simulink model "TV_render_car"  (R2025b)
settings: Solver=VariableStepAuto  StartTime=0.0  StopTime=90  MaxStep=0.03  RelTol=1e-3
libraries: simulink x4, vehdynlibsteering x1, sim3dlib x1, sim3dautolib x1, slpidlib x1, autolibshared x1
settings Model: Creator=Utente  LastModifiedBy=Utente

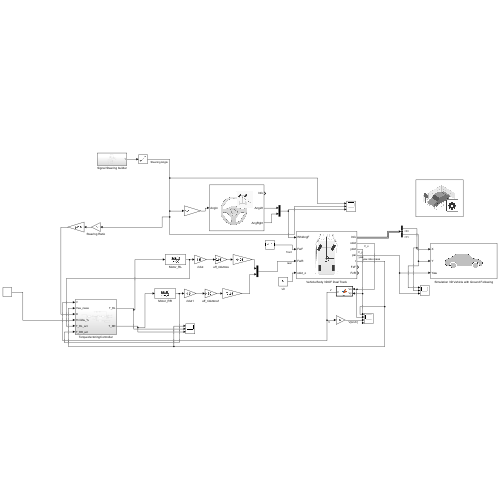
[thumbnail: Simulink's stored preview of the top-level diagram]
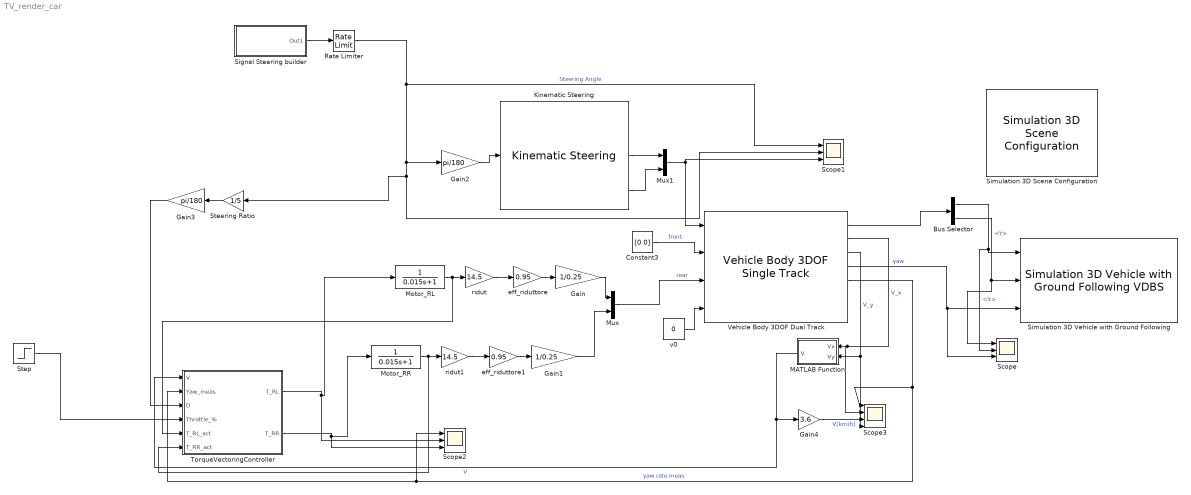
== system TV_render_car ==
  Bus Selector : BusSelector  OutputSignals=InertFrm.Geom.Disp.X,InertFrm.Geom.Disp.Y
  Constant3 : Constant  Value=[0 0]
  Gain : Gain  Gain=1/0.25
  Gain1 : Gain  Gain=1/0.25
  Gain2 : Gain  Gain=pi/180
  Gain3 : Gain  Gain=pi/180
  Gain4 : Gain  Gain=3.6
  Kinematic Steering : vehdynlibsteering/Kinematic Steering  StrgType=Ackerman  StrgRatioType=Constant  Loc=Front  NrmlFctr=0.01  TrckWdth=1.2  WhlBase=1.55  Db=0  StrgRng=pi  StrgAngBpts="[-6.2832   -5.0265   -3.7699   -2.5133   -1.2566         0    1.2566    2.5133    3.7699    5.0265    6.2832]"  StrgRatioTbl=|  StrgRatio=5  PctAckIn=off  PctAck=100  PctAckTbl=ones(1,11)*100  StrgArmLngth=0.1  RckCsLngth=0.5  TieRodLngth=0.248  D=0.2  PnnRadius=0.00085818  PnnRadiusTbl="[0.0055    0.0055    0.0056    0.0057    0.0058    0.0057    0.0057    0.0057    0.0056    0.0055    0.0055]"  RodLngth=0.1  ParaArmLngth=0.9  aMode=2
      | [13.5000   13.3750   13.2500   13.1250   13.0000   13.0000   13.0000   13.1250   13.2500   13.3750   13.5000
      | ]
  MATLAB Function : MATLAB Function  TreatAsAtomicUnit=on
  Motor_RL : TransferFcn  Denominator=[0.015 1]
  Motor_RR : TransferFcn  Denominator=[0.015 1]
  Mux : Mux  Inputs=2
  Mux1 : Mux  Inputs=2
  Rate Limiter : RateLimiter  RisingSlewLimit=300  FallingSlewLimit=-300  SampleTimeMode=inherited
  Scope : Scope  NumInputPorts=3
      settings: ActiveDisplayYMinimum=-522.68712025168293  ActiveDisplayYMaximum=261.84287437072271
  Scope1 : Scope  NumInputPorts=3
      settings: ActiveDisplayYMinimum=-50  ActiveDisplayYMaximum=50
  Scope2 : Scope  NumInputPorts=3
      settings: ActiveDisplayYMinimum=-1.4348752582042583  ActiveDisplayYMaximum=1.2936169370543145  DataLoggingVariableName=ScopeData2
  Scope3 : Scope  NumInputPorts=4
      settings: ActiveDisplayYMinimum=-15.9041702308022  ActiveDisplayYMaximum=143.13753207721982  DataLoggingVariableName=ScopeData3
  Signal Steering builder : Subsystem
  Simulation 3D Scene Configuration : sim3dlib/Simulation 3D Scene Configuration  Priority=0  ProjectFormat=Default Scenes  SceneDesc=Double lane change  ProjectName=Z:\.Programmi\MATLAB\toolbox\shared\sim3d_projects\automotive_project_windows\UE\WindowsNoEditor\VehicleSimulation.exe  ScenePath=/Game/Maps/HwStrght  EnableOpenDRIVE=off  vehTagList={'Custom';'Scene Origin';'SimulinkVehicle1'}  vehTag=SimulinkVehicle1  AttachedCameraRelativeTranslation=[0 0 0]  FreeCameraDefaultInitialTranslation=[-6, 0, 2]  AttachedCameraRelativeRotation=[0 0 0]  FreeCameraDefaultInitialRotation=[0, -15, 0]  ViewpointName=Custom  FreeCameraInitialTranslation=[0 0 0]  ViewpointTranslation=[0 0 0]  FreeCameraInitialRotation=[0 0 0]  ViewpointRotation=[0 0 0]  OpVisEn=off  Ts=.02  EnableWindow=on  EnableRemoteAccess=off  EnableWeather=off  SunAzimuth=90  SunAltitude=40.0  EnableGeospatialSun=off  Latitude=0  Longitude=0  Date=2023-01-01  Time=10:30:00  GeoTimeZone=-5.0  SunDaylightSaving=off  wind=1  clouds=10  EnableVolumetricClouds=off  CloudCoverage=0  CloudAltitude=6  fog=0  rain=0  RaindropsEffect=off  SnowDensity=0  EnableGeospatial=off  TilesetSource=Earth terrain  UseTrueOrigin=off  OriginHeight=200  OriginLatitude=40.744652  OriginLongitude=-73.988864  MapStyle=Aerial  AdditionalAssetIDs=[]  UseAdvancedSunSky=off  SolarTime=11  TimeZone=-5  Day=21  Month=9  Year=2022  UseDaylightSavingTime=on  DSTStartDay=10  DSTStartMonth=3  DSTEndDay=3  DSTEndMonth=11  DSTSwitchHour=2  sensorTag=MainCamera1  sensorId=1  sensorName=MainCamera1  mountLoc=Origin  offsetFlag=off  tmountOffset=[0, 0, 0]  rmountOffset=[0, 0, 0]  HorizontalResolution=1280  VerticalResolution=720  HorizontalFOV=60  mountPoint=[0 0 0]  mountOrientation=[0 0 0]  aMode=2  ID=1  GeoTrigger=Inactive  ViewNameList={'Custom'}  ViewTranslationList={'[0 0 0]'}  ViewRotationList={'[0 0 0]'}
      settings: LibrarySourceBlock=vehdynlibsim3dcore/Simulation 3D Scene Configuration
  Simulation 3D Vehicle with Ground Following : sim3dautolib/Simulation 3D Vehicle with Ground Following VDBS  Priority=-1  PassVehMesh=Formula student vehicle  MeshPath=/MathWorksAutomotiveContent/Vehicles/Muscle/Meshes/SK_MuscleCar.SK_MuscleCar  TrackWidth=1.9  WheelBase=3  WheelRadius=0.35  VehColor=Red  CoordinateSystem=SAE  InitialPos=[0, 0, 0]  InitialRot=[0,0,0]  ActorName=SimulinkVehicle1  VehLightsControl=off  HeadlightColor=[ 1, 1, 1 ]  HighBeamIntensity=100000  LowBeamIntensity=60000  HighBeamConeAngle=1.22  LowBeamConeAngle=1.22  LeftHeadlightOrientation=[ 0, 0 ]  RightHeadlightOrientation=[ 0, 0 ]  BrakelightIntensity=200  ReverselightIntensity=500  SignallightIntensity=500  SignallightPeriod=1  SignalPulseWidth=50  SampleTime=-1  ActorType=SimulinkVehicle  ID=1  aMode=2  ActorTag=SimulinkVehicle1  CoordinateScheme=0
      settings: LibrarySourceBlock=vehdynlibsim3d/Simulation 3D Vehicle with Ground Following
  Steering Ratio : Gain  Gain=1/5
  Step : Step  Time=2  After=50  SampleTime=0
  TorqueVectoringController : Subsystem
  Vehicle Body 3DOF Dual Track : autolibshared/Vehicle Body 3DOF Single Track  trackMode=Dual  inputMode=External longitudinal forces  frontSteerMode=on  rearSteerMode=off  windMode=off  muMode=off  extFMode=off  extMMode=off  htchFMode=off  htchMMode=off  extXo=off  extpsio=off  extxdoto=on  extro=off  extYo=off  extTamb=off  extydoto=off  aMode=2  NF=2  NR=2  m=320  a=0.775  b=0.775  h=0.35  dh=1  hh=0.2  X_o=0  xdot_o=0  CalphaMode=off  sigmaMode=on  d=0  hl=0  w=[1.2,1.2]  Cy_f=35e3  Cy_r=45e3  sigma_f=.1  sigma_r=.1  alpha_f_brk=[-0.785, -0.628, -0.471, -0.314, -0.157, 0.000, 0.157, 0.314, 0.471, 0.628, 0.785]  Cy_f_data=[2000, 3000, 4000, 5500, 7000, 9000, 7000, 5500, 4000, 3000, 2000]  alpha_r_brk=[-0.785, -0.628, -0.471, -0.314, -0.157, 0.000, 0.157, 0.314, 0.471, 0.628, 0.785]  Cy_r_data=[2000, 3000, 4000, 5500, 7000, 9000, 7000, 5500, 4000, 3000, 2000]  Y_o=5  ydot_o=0  Izz=200  psi_o=0  r_o=0  Af=1.1  Cd=1.3  Cl=-1  Cpm=.1  beta_w=[0 0.01:0.01:0.3]  Cs=[0:0.03:0.9]  Cym=[0 1e-6:0.01:0.3]  Pabs=101325  Tair=273  g=9.81  mu=1  xdot_tol=.01  Fznom=2400  Fxtire_sat=7e4  Fytire_sat=7e4  longOff=0  latOff=0  vertOff=0  wrapAng=off
      settings: LibrarySourceBlock=vehdynlibeom/Vehicle Body 3DOF Dual Track
  eff_riduttore : Gain  Gain=0.95
  eff_riduttore1 : Gain  Gain=0.95
  ridut : Gain  Gain=14.5
  ridut1 : Gain  Gain=14.5
  v0 : Constant  Value=0
  wires:
  Constant3/1 -> Vehicle Body 3DOF Dual Track/2  "front"
  Mux/1 -> Vehicle Body 3DOF Dual Track/3  "rear"
  Gain/1 -> Mux/1
  Gain1/1 -> Mux/2
  Kinematic Steering/2 -> Mux1/1
  Kinematic Steering/3 -> Mux1/2
  Mux1/1 -> Vehicle Body 3DOF Dual Track/1, Scope1/3
  Gain2/1 -> Kinematic Steering/1
  Vehicle Body 3DOF Dual Track/2 -> Scope3/2, MATLAB Function/1(Vx)  "V_x"
  Vehicle Body 3DOF Dual Track/3 -> Scope3/4, MATLAB Function/2(Vy)  "V_y"
  Bus Selector/1 -> Scope/2, Simulation 3D Vehicle with Ground Following/1  "<X>"
  Bus Selector/2 -> Scope/1, Simulation 3D Vehicle with Ground Following/2  "<Y>"
  Vehicle Body 3DOF Dual Track/5 -> Scope2/1, TorqueVectoringController/2(Yaw_meas), Scope3/1  "yaw rate meas"
  v0/1 -> Vehicle Body 3DOF Dual Track/4
  Vehicle Body 3DOF Dual Track/1 -> Bus Selector/1
  Motor_RL/1 -> TorqueVectoringController/5(T_RL_act), ridut/1
  eff_riduttore/1 -> Gain/1
  ridut/1 -> eff_riduttore/1
  Motor_RR/1 -> TorqueVectoringController/6(T_RR_act), ridut1/1
  ridut1/1 -> eff_riduttore1/1
  eff_riduttore1/1 -> Gain1/1
  Steering Ratio/1 -> Gain3/1
  Gain3/1 -> TorqueVectoringController/3(D)
  Step/1 -> TorqueVectoringController/4(Throttle_%)
  MATLAB Function/1(V) -> TorqueVectoringController/1(V), Gain4/1  "V"
  Vehicle Body 3DOF Dual Track/4 -> Scope/3, Simulation 3D Vehicle with Ground Following/3  "yaw"
  Signal Steering builder/1(Out1) -> Rate Limiter/1
  TorqueVectoringController/1(T_RL) -> Scope2/2, Motor_RL/1
  TorqueVectoringController/2(T_RR) -> Scope2/3, Motor_RR/1
  Gain4/1 -> Scope3/3  "V[km/h]"
  Rate Limiter/1 -> Steering Ratio/1, Scope1/2, Gain2/1, Scope1/1  "Steering Angle"

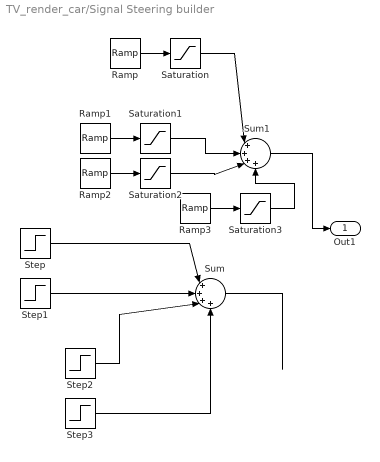
== system TV_render_car/Signal Steering builder ==
  Ramp : simulink/Sources/Ramp  slope=20  start=0  InitialOutput=0
  Ramp1 : simulink/Sources/Ramp  slope=-20  start=14  InitialOutput=0
  Ramp2 : simulink/Sources/Ramp  slope=-20  start=14  InitialOutput=0
  Ramp3 : simulink/Sources/Ramp  slope=20  start=22  InitialOutput=0
  Saturation{,1..3} (4 alike) : Saturate  UpperLimit=40  LowerLimit=-40
  Step : Step  Time=6  After=50  SampleTime=0
  Step1 : Step  Time=14  After=-50  SampleTime=0
  Step2 : Step  Time=14  After=-50  SampleTime=0
  Step3 : Step  Time=22  After=50  SampleTime=0
  Sum : Sum  Inputs=|++++
  Sum1 : Sum  Inputs=|++++
  Out1 : Outport
  wires:
  Step/1 -> Sum/1
  Step1/1 -> Sum/2
  Step3/1 -> Sum/4
  Step2/1 -> Sum/3
  Sum/1 -> ?
  Ramp/1 -> Saturation/1
  Ramp1/1 -> Saturation1/1
  Ramp2/1 -> Saturation2/1
  Ramp3/1 -> Saturation3/1
  Saturation3/1 -> Sum1/4
  Saturation/1 -> Sum1/1
  Saturation1/1 -> Sum1/2
  Saturation2/1 -> Sum1/3
  Sum1/1 -> Out1/1

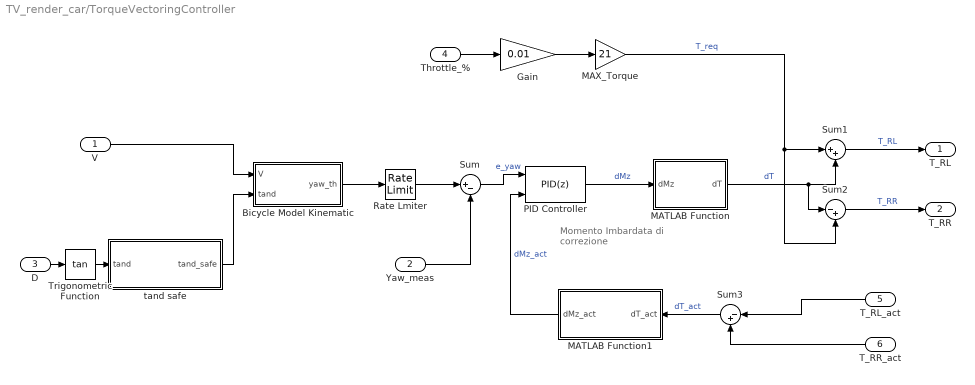
== system TV_render_car/TorqueVectoringController ==
  note: Momento Imbardata di correzione
  V : Inport
  Yaw_meas : Inport  Port=2
  D : Inport  Port=3
  Throttle_% : Inport  Port=4
  T_RL_act : Inport  Port=5
  T_RR_act : Inport  Port=6
  Bicycle Model Kinematic : MATLAB Function  TreatAsAtomicUnit=on
  Gain : Gain  Gain=0.01
  MATLAB Function : MATLAB Function  TreatAsAtomicUnit=on
  MATLAB Function1 : MATLAB Function  TreatAsAtomicUnit=on
  MAX_Torque : Gain  Gain=21
  PID Controller : slpidlib/PID Controller  Controller=PID  Form=Parallel  TimeDomain=Discrete-time  UseExternalTs=off  SampleTime=0.05  IntegratorMethod=Forward Euler  FilterMethod=Forward Euler  ControllerParametersSource=internal  P=50  I=0.01  UseKiTs=off  D=0  UseExternalDerivativeSource=off  N=100  UseFilter=on  TunerSelectOption=Transfer Function Based (PID Tuner App)  InitialConditionSource=internal  InitialConditionForIntegrator=0  InitialConditionForFilter=0  DifferentiatorICPrevScaledInput=0  ExternalReset=none  TrackingMode=on  Kt=0.7  LimitOutput=on  SatLimitsSource=internal  UpperSaturationLimit=10  LowerSaturationLimit=-10  LinearizeAsGain=on  AntiWindupMode=none  Kb=1  LimitIntegrator=off  UpperIntegratorSaturationLimit=inf  LowerIntegratorSaturationLimit=-inf  POutMin=[]  POutMax=[]  IOutMin=[]  IOutMax=[]  DOutMin=[]  DOutMax=[]  NOutMin=[]  NOutMax=[]  SumOutMin=[]  SumOutMax=[]  SaturationOutMin=[]  SaturationOutMax=[]  PParamMin=[]  PParamMax=[]  IParamMin=[]  IParamMax=[]  DParamMin=[]  DParamMax=[]  NParamMin=[]  NParamMax=[]  KbParamMin=[]  KbParamMax=[]  KtParamMin=[]  KtParamMax=[]  KbOutMin=[]  KbOutMax=[]  KtOutMin=[]  KtOutMax=[]  IntegratorOutMin=[]  IntegratorOutMax=[]  FilterOutMin=[]  FilterOutMax=[]  SumI1OutMin=[]  SumI1OutMax=[]  SumI2OutMin=[]  SumI2OutMax=[]  SumI3OutMin=[]  SumI3OutMax=[]  SumI4OutMin=[]  SumI4OutMax=[]  SumDOutMin=[]  SumDOutMax=[]  DifferentiatorOutMin=[]  DifferentiatorOutMax=[]  FilterDiffOutCoefMin=[]  FilterDiffOutCoefMax=[]  ReciprocalOutMin=[]  ReciprocalOutMax=[]  SumDenOutMin=[]  SumDenOutMax=[]  SumNumOutMin=[]  SumNumOutMax=[]  DivideOutMin=[]  DivideOutMax=[]  UdiffTsProdOutMin=[]  UdiffTsProdOutMax=[]  NTsProdOutMin=[]  NTsProdOutMax=[]  UintegralTsProdOutMin=[]  UintegralTsProdOutMax=[]  UngainTsProdOutMin=[]  UngainTsProdOutMax=[]  ClampingZeroOutDataTypeStr=Inherit: Inherit via back propagation  ClampingZeroOutMin=[]  ClampingZeroOutMax=[]  FilterDenConstantOutDataTypeStr=Inherit: Inherit via back propagation  FilterDenConstantOutMin=[]  FilterDenConstantOutMax=[]  PCopyOutDataTypeStr=Inherit: Inherit via back propagation  PCopyOutMin=[]  PCopyOutMax=[]  NCopyOutDataTypeStr=Inherit: Inherit via back propagation  NCopyOutMin=[]  NCopyOutMax=[]  IntegratorContinuousStateAttributes=''  IntegratorStateMustResolveToSignalObject=off  IntegratorRTWStateStorageClass=Auto  FilterContinuousStateAttributes=''  FilterStateMustResolveToSignalObject=off  FilterRTWStateStorageClass=Auto  ParallelPVariant=InternalParameters  IdealPVariant=Disabled  IVariant=InternalParameters  DVariant=InternalParameters  IntegratorVariant=Discrete  SatVariant=Enabled  AWVariant=Passthrough  PCopyVariant=Disabled  TRVariant=Enabled  FdbkBlocksVariant=Forward  IdealPFdbkVariant=Disabled  SatFdbkVariant=Disabled  DerivativeFilterVariant=ForwardEulerFilter  NVariant=InternalParameters  NCopyVariant=Disabled  FilterICVariant=InternalICsFilter  IntegratorICVariant=InternalICs  ExternalResetVariant=Disabled  TRSumVariant=TrackingMode  SumFdbkVariant=Disabled  SumVariant=Sum_PID  TsampFilterVariant=InternalTs  TsampNgainVariant=Passthrough  TsampIntegralVariant=Disabled_SignalSpec  ExternalSaturationOutDataTypeStr=Inherit: Same as second input  DerivativeSourceVariant=ErrorSignal  PreIntVariant=InternalPreInt
  Rate Lmiter : RateLimiter  RisingSlewLimit=0.5  FallingSlewLimit=-0.5  SampleTimeMode=inherited
  Sum : Sum  Inputs=|+-
  Sum1 : Sum  Inputs=|++
  Sum2 : Sum  Inputs=|-+
  Sum3 : Sum  Inputs=|-+
  Trigonometric Function : Trigonometry  Operator=tan
  tand safe : MATLAB Function  TreatAsAtomicUnit=on
  T_RL : Outport
  T_RR : Outport  Port=2
  wires:
  Throttle_%/1 -> Gain/1
  Trigonometric Function/1 -> tand safe/1(tand)
  D/1 -> Trigonometric Function/1
  tand safe/1(tand_safe) -> Bicycle Model Kinematic/2(tand)
  V/1 -> Bicycle Model Kinematic/1(V)
  Yaw_meas/1 -> Sum/2
  Sum/1 -> PID Controller/1  "e_yaw"
  PID Controller/1 -> MATLAB Function/1(dMz)  "dMz"
  MAX_Torque/1 -> Sum2/2, Sum1/1  "T_req"
  Sum1/1 -> T_RL/1  "T_RL"
  MATLAB Function/1(dT) -> Sum2/1, Sum1/2  "dT"
  Sum2/1 -> T_RR/1  "T_RR"
  Sum3/1 -> MATLAB Function1/1(dT_act)  "dT_act"
  MATLAB Function1/1(dMz_act) -> PID Controller/2  "dMz_act"
  Gain/1 -> MAX_Torque/1
  T_RL_act/1 -> Sum3/1
  T_RR_act/1 -> Sum3/2
  Bicycle Model Kinematic/1(yaw_th) -> Rate Lmiter/1
  Rate Lmiter/1 -> Sum/1

== matlab function TV_render_car/TorqueVectoringController/Bicycle Model Kinematic ==
  data: V input; yaw_th output; tand input
function yaw_th = fcn(V,tand)
L = 1.55; %passo veicolo [m]
yaw_th = (V / L) * tand;

== matlab function TV_render_car/TorqueVectoringController/MATLAB Function1 ==
  data: dT_act input; dMz_act output
function dMz_act = fcn(dT_act)
Rw = 0.2; %raggio ruota [m]
w  = 1.2; %carreggiata [m]

dMz_act = dT_act * w / (2*Rw);

== matlab function TV_render_car/MATLAB Function ==
  data: Vx input; V output; Vy input
function V = fcn(Vx,Vy)

V = (Vx^2 + Vy^2)^0.5;

== matlab function TV_render_car/TorqueVectoringController/tand safe ==
  data: tand input; tand_safe output
% function tand_safe = fcn(tand)
%     tand_safe = sign(tand) * max(abs(tand), tan(2*pi/180));
% end

function tand_safe = fcn(tand)
    soglia = tan(5*pi/180);  % 5° 
    
    if abs(tand) < soglia
        tand_safe = 0;  % TV disattivato sotto soglia
    else
        tand_safe = tand;  % passa il valore reale senza clamp
    end
end

== matlab function TV_render_car/TorqueVectoringController/MATLAB Function ==
  data: dMz input; dT output
function dT = fcn(dMz)
Rw = 0.2; %raggio ruota [m]
w  = 1.2; %carreggiata [m]

dT = dMz * Rw / w;
